simulink model "drembao_vel_torq"  (R2020b)
settings: Solver=VariableStepAuto  StartTime=0.0  StopTime=0.7998  FixedStep=dt  RelTol=1e-10  AbsTol=1e-14
values from neighbouring files (symbols this model uses):
  flux_initial = [1; 1]    [spmsm_param.m]    (also in spmsm_param_exp.m)
  G = [gamma, 0; 0, gamma]    [spmsm_param.m]    (also in spmsm_param_exp.m)
  gamma = 0.01    [spmsm_param.m]    (also in spmsm_param_exp.m = 50)
  gamma_L = 20000    [spmsm_param.m]    (also in spmsm_param_exp.m = 10000)
  gamma_w = 30000    [spmsm_param.m]    (also in spmsm_param_exp.m = 10000)
  I_d = 1    [spmsm_param.m]
  I_q = 1    [spmsm_param.m]
  I_w = 50    [spmsm_param.m]
  J = 59e-6    (= 5.9e-05)    [spmsm_param.m]    (also in spmsm_param_exp.m = 0.0015)
  L = 40.03e-3    (= 0.04003)    [spmsm_param.m]    (also in spmsm_param_exp.m = 0.0014)
  lm = 0.2086    [spmsm_param.m]    (also in spmsm_param_exp.m = 0.032)
  mu = 800    [spmsm_param.m]    (also in spmsm_param_exp.m = 100)
  np = 5    [spmsm_param.m]    (also in spmsm_param_exp.m = 8)
  nu = [50, 550]    [spmsm_param.m]    (also in spmsm_param_exp.m)
  P_d = 5    [spmsm_param.m]
  P_q = 5    [spmsm_param.m]
  P_w = 0.4    [spmsm_param.m]
  R = 8.875    [spmsm_param.m]    (also in spmsm_param_exp.m = 0.39)
  rho_1 = 0.9    [spmsm_param.m]    (also in spmsm_param_exp.m)
  S = [0, -1; 1, 0]    [spmsm_param.m]    (also in spmsm_param_exp.m)
  T = 2.0000e-04    (= 0.0002)    [prepare_timeseries_from_csv.m]
undefined symbols (not defined in the file or in its folder): j
libraries: pid_lib x3
settings Model: Creator=root  LastModifiedBy=R-1221
settings DataIOCC: ReturnWorkspaceOutputs=off
settings DebuggingCC: ArithmeticOperatorsInVariantConditions=warning
settings SFSimCC: SimUseLocalCustomCode=off  CustomCodeUndefinedFunction=UseInterfaceOnly
settings RTWCC: RTWUseLocalCustomCode=off

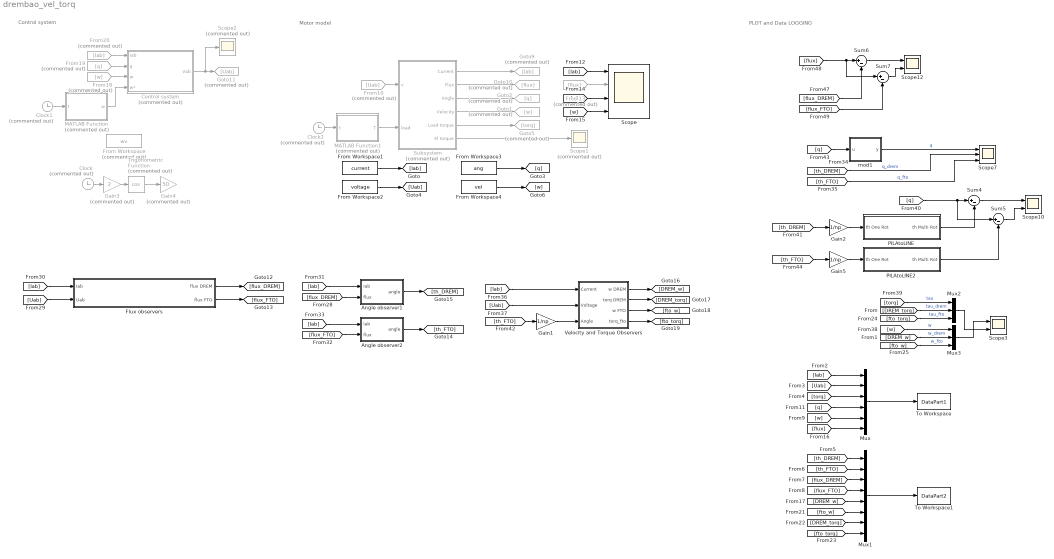
== system drembao_vel_torq ==
  note: PLOT and Data LOGGING
  note: Control system
  note: Motor model
  Angle observer1 : Subsystem
  Angle observer2 : Subsystem
  Clock : Clock  Commented=on
  Clock1 : Clock  Commented=on
  Clock2 : Clock  Commented=on
  Control system : Subsystem  Commented=on
  Flux observers : Subsystem
  From Workspace : FromWorkspace  Commented=on  VariableName=wv  SampleTime=-1
  From Workspace1 : FromWorkspace  VariableName=current  SampleTime=T
  From Workspace2 : FromWorkspace  VariableName=voltage  SampleTime=T
  From Workspace3 : FromWorkspace  VariableName=ang  SampleTime=T
  From Workspace4 : FromWorkspace  VariableName=vel  SampleTime=T
  From10 : From  Commented=on  GotoTag=Uab
  From13 : From  Commented=on  GotoTag=flux
  From18 : From  Commented=on  GotoTag=w
  From19 : From  Commented=on  GotoTag=q
  From20 : From  Commented=on  GotoTag=Iab
  Gain1 : Gain  Gain=1/np
  Gain2 : Gain  Gain=1/np
  Gain3 : Gain  Commented=on  Gain=2
  Gain4 : Gain  Commented=on  Gain=50
  Gain5 : Gain  Gain=1/np
  Goto1 : Goto  Commented=on  GotoTag=w
  Goto10 : Goto  Commented=on  GotoTag=flux
  Goto11 : Goto  Commented=on  GotoTag=Uab
  Goto2 : Goto  Commented=on  GotoTag=q
  Goto5 : Goto  Commented=on  GotoTag=torq
  Goto9 : Goto  Commented=on  GotoTag=Iab
  MATLAB Function : MATLAB Function  Commented=on  TreatAsAtomicUnit=on
  MATLAB Function1 : MATLAB Function  Commented=on  TreatAsAtomicUnit=on
  Mux : Mux  Inputs=6
  Mux1 : Mux  Inputs=8
  Mux2 : Mux  Inputs=3
  Mux3 : Mux  Inputs=3
  PILAtoLINE : Subsystem
  PILAtoLINE2 : Subsystem
  Scope : Scope  NumInputPorts=4
  Scope1 : Scope  Commented=on
  Scope10 : Scope  NumInputPorts=2
  Scope12 : Scope  NumInputPorts=2
  Scope2 : Scope  Commented=on
  Scope3 : Scope  NumInputPorts=2
  Scope7 : Scope  NumInputPorts=3
  Subsystem : Subsystem  Commented=on
  Sum{4..7} (4 alike) : Sum  Inputs=|+-
  To Workspace : ToWorkspace  VariableName=DataPart1  SaveFormat=Timeseries  SampleTime=-1
  To Workspace1 : ToWorkspace  VariableName=DataPart2  SaveFormat=Timeseries  SampleTime=-1
  Trigonometric Function : Trigonometry  Commented=on  Operator=cos
  Velocity and Torque Observers : Subsystem
  mod1 : MATLAB Function  TreatAsAtomicUnit=on
  wires:
  Subsystem/5(Load torque) -> Goto5/1
  Subsystem/2(Flux) -> Goto10/1
  Subsystem/1(Current) -> Goto9/1
  Subsystem/4(Velocity) -> Goto1/1
  Subsystem/3(Angle) -> Goto2/1
  Subsystem/6(El torque) -> Scope1/1
  From10/1 -> Subsystem/1(v)
  [Iab] -> Scope/1
  From13/1 -> Scope/2
  [q] -> Scope/3
  [w] -> Scope/4
  From18/1 -> Control system/3(w)
  MATLAB Function/1(w) -> Control system/4(w*)
  From19/1 -> Control system/2(q)
  From20/1 -> Control system/1(Iab)
  MATLAB Function1/1(T) -> Subsystem/2(load)
  Sum6/1 -> Scope12/1
  [flux] -> Sum7/1, Sum6/1
  [flux_DREM] -> Sum6/2
  [flux_FTO] -> Sum7/2
  Sum7/1 -> Scope12/2
  [Uab] -> Flux observers/2(Uab)
  [Iab] -> Flux observers/1(Iab)
  Flux observers/1(flux DREM) -> [flux_DREM]
  Flux observers/2(flux FTO) -> [flux_FTO]
  [q] -> mod1/1(u)
  [flux_DREM] -> Angle observer1/2(flux)
  [Iab] -> Angle observer1/1(Iab)
  Angle observer1/1(angle) -> [th_DREM]
  [Iab] -> Angle observer2/1(Iab)
  [flux_FTO] -> Angle observer2/2(flux)
  [th_FTO] -> Scope7/3  "q_fto"
  PILAtoLINE/1(th Multi Rot) -> Sum4/2
  [th_DREM] -> Gain2/1
  mod1/1(y) -> Scope7/1  "q"
  [th_DREM] -> Scope7/2  "q_drem"
  Angle observer2/1(angle) -> [th_FTO]
  [Uab] -> Velocity and Torque Observers/2(Voltage)
  Gain1/1 -> Velocity and Torque Observers/3(Angle)
  Velocity and Torque Observers/4(torq_fto) -> [fto_torq]
  [Iab] -> Velocity and Torque Observers/1(Current)
  Velocity and Torque Observers/3(w FTO) -> [fto_w]
  Velocity and Torque Observers/1(w DREM) -> [DREM_w]
  Velocity and Torque Observers/2(torq DREM) -> [DREM_torq]
  [th_FTO] -> Gain1/1
  Gain2/1 -> PILAtoLINE/1(th One Rot)
  [q] -> Sum5/1, Sum4/1
  Sum4/1 -> Scope10/1
  [th_FTO] -> Gain5/1
  Gain5/1 -> PILAtoLINE2/1(th One Rot)
  PILAtoLINE2/1(th Multi Rot) -> Sum5/2
  Sum5/1 -> Scope10/2
  Clock/1 -> Gain3/1
  Gain3/1 -> Trigonometric Function/1
  Trigonometric Function/1 -> Gain4/1
  [w] -> Mux3/1  "w"
  [DREM_w] -> Mux3/2  "w_drem"
  [DREM_torq] -> Mux2/2  "tau_drem"
  [torq] -> Mux2/1  "tau"
  [Iab] -> Mux/1
  [Uab] -> Mux/2
  [torq] -> Mux/3
  Mux/1 -> To Workspace/1
  [th_DREM] -> Mux1/1
  [th_FTO] -> Mux1/2
  [flux_DREM] -> Mux1/3
  [flux_FTO] -> Mux1/4
  Mux1/1 -> To Workspace1/1
  [q] -> Mux/4
  [w] -> Mux/5
  [flux] -> Mux/6
  [DREM_torq] -> Mux1/7
  [fto_w] -> Mux1/6
  [DREM_w] -> Mux1/5
  [fto_torq] -> Mux1/8
  Control system/1(Vab) -> Scope2/1, Goto11/1
  Clock1/1 -> MATLAB Function/1(t)
  Clock2/1 -> MATLAB Function1/1(t)
  From Workspace1/1 -> [Iab]
  From Workspace2/1 -> [Uab]
  From Workspace4/1 -> [w]
  From Workspace3/1 -> [q]
  [fto_torq] -> Mux2/3  "tau_fto"
  [fto_w] -> Mux3/3  "w_fto"
  Mux3/1 -> Scope3/1
  Mux2/1 -> Scope3/2

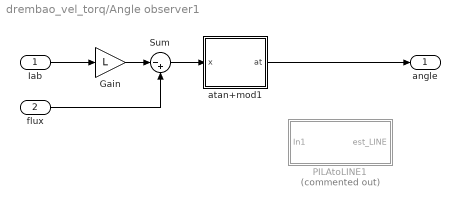
== system drembao_vel_torq/Angle observer1 ==
  Iab : Inport
  flux : Inport  Port=2
  Gain : Gain  Gain=L
  PILAtoLINE1 : Subsystem  Commented=on
  Sum : Sum  Inputs=|-+
  atan+mod1 : MATLAB Function  TreatAsAtomicUnit=on
  angle : Outport  VectorParamsAs1DForOutWhenUnconnected=off
  wires:
  Iab/1 -> Gain/1
  Gain/1 -> Sum/1
  flux/1 -> Sum/2
  Sum/1 -> atan+mod1/1(x)
  atan+mod1/1(at) -> angle/1

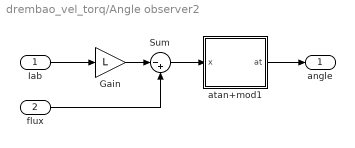
== system drembao_vel_torq/Angle observer2 ==
  Iab : Inport
  flux : Inport  Port=2
  Gain : Gain  Gain=L
  Sum : Sum  Inputs=|-+
  atan+mod1 : MATLAB Function  TreatAsAtomicUnit=on
  angle : Outport  VectorParamsAs1DForOutWhenUnconnected=off
  wires:
  Iab/1 -> Gain/1
  Gain/1 -> Sum/1
  flux/1 -> Sum/2
  Sum/1 -> atan+mod1/1(x)
  atan+mod1/1(at) -> angle/1

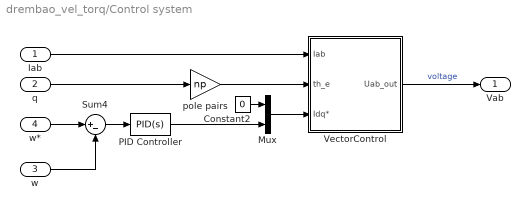
== system drembao_vel_torq/Control system ==
  Iab : Inport  PortDimensions=[2, 1]
  q : Inport  Port=2
  w : Inport  Port=3
  w* : Inport  Port=4
  Constant2 : Constant  Value=0
  Mux : Mux  Inputs=2
  PID Controller : pid_lib/PID Controller  Controller=PID  Form=Parallel  TimeDomain=Continuous-time  UseExternalTs=off  SampleTime=-1  IntegratorMethod=Forward Euler  FilterMethod=Forward Euler  ControllerParametersSource=internal  P=P_w  I=I_w  D=0  UseFilter=on  N=100  TunerSelectOption=Transfer Function Based (PID Tuner App)  InitialConditionSource=internal  InitialConditionForIntegrator=0  InitialConditionForFilter=0  DifferentiatorICPrevScaledInput=0  ExternalReset=none  TrackingMode=off  Kt=1  LimitOutput=off  SatLimitsSource=internal  UpperSaturationLimit=inf  LowerSaturationLimit=-inf  LinearizeAsGain=on  AntiWindupMode=none  Kb=1  POutMin=[]  POutMax=[]  IOutMin=[]  IOutMax=[]  DOutMin=[]  DOutMax=[]  NOutMin=[]  NOutMax=[]  SumOutMin=[]  SumOutMax=[]  SaturationOutMin=[]  SaturationOutMax=[]  PParamMin=[]  PParamMax=[]  IParamMin=[]  IParamMax=[]  DParamMin=[]  DParamMax=[]  NParamMin=[]  NParamMax=[]  KbParamMin=[]  KbParamMax=[]  KtParamMin=[]  KtParamMax=[]  KbOutMin=[]  KbOutMax=[]  KtOutMin=[]  KtOutMax=[]  IntegratorOutMin=[]  IntegratorOutMax=[]  FilterOutMin=[]  FilterOutMax=[]  SumI1OutMin=[]  SumI1OutMax=[]  SumI2OutMin=[]  SumI2OutMax=[]  SumI3OutMin=[]  SumI3OutMax=[]  SumI4OutMin=[]  SumI4OutMax=[]  SumDOutMin=[]  SumDOutMax=[]  DifferentiatorOutMin=[]  DifferentiatorOutMax=[]  FilterDiffOutCoefMin=[]  FilterDiffOutCoefMax=[]  ReciprocalOutMin=[]  ReciprocalOutMax=[]  SumDenOutMin=[]  SumDenOutMax=[]  SumNumOutMin=[]  SumNumOutMax=[]  DivideOutMin=[]  DivideOutMax=[]  UdiffTsProdOutMin=[]  UdiffTsProdOutMax=[]  NTsProdOutMin=[]  NTsProdOutMax=[]  UintegralTsProdOutMin=[]  UintegralTsProdOutMax=[]  UngainTsProdOutMin=[]  UngainTsProdOutMax=[]  IntegratorContinuousStateAttributes=''  IntegratorStateMustResolveToSignalObject=off  IntegratorRTWStateStorageClass=Auto  FilterContinuousStateAttributes=''  FilterStateMustResolveToSignalObject=off  FilterRTWStateStorageClass=Auto  ParallelPVariant=InternalParameters  IdealPVariant=Disabled  IVariant=InternalParameters  DVariant=InternalParameters  IntegratorVariant=Continuous  SatVariant=Disabled  AWVariant=Passthrough  PCopyVariant=Disabled  TRVariant=Disabled  FdbkBlocksVariant=Forward  IdealPFdbkVariant=Disabled  SatFdbkVariant=Disabled  DerivativeFilterVariant=ContFilter  NVariant=InternalParameters  NCopyVariant=Disabled  FilterICVariant=InternalICsFilter  IntegratorICVariant=InternalICs  ExternalResetVariant=Disabled  TRSumVariant=Passthrough  SumFdbkVariant=Disabled  SumVariant=Sum_PID  TsampFilterVariant=InternalTs  TsampNgainVariant=Passthrough  TsampIntegralVariant=Passthrough  ExternalSaturationOutDataTypeStr=Inherit: Same as second input
  Sum4 : Sum  Inputs=|+-
  VectorControl : Subsystem
  pole pairs : Gain  Gain=np
  Vab : Outport  PortDimensions=[2, 1]  VectorParamsAs1DForOutWhenUnconnected=off
  wires:
  w*/1 -> Sum4/1
  VectorControl/1(Uab_out) -> Vab/1  "voltage"
  w/1 -> Sum4/2
  Iab/1 -> VectorControl/1(Iab)
  Sum4/1 -> PID Controller/1
  q/1 -> pole pairs/1
  pole pairs/1 -> VectorControl/2(th_e)
  Mux/1 -> VectorControl/3(Idq*)
  PID Controller/1 -> Mux/2
  Constant2/1 -> Mux/1

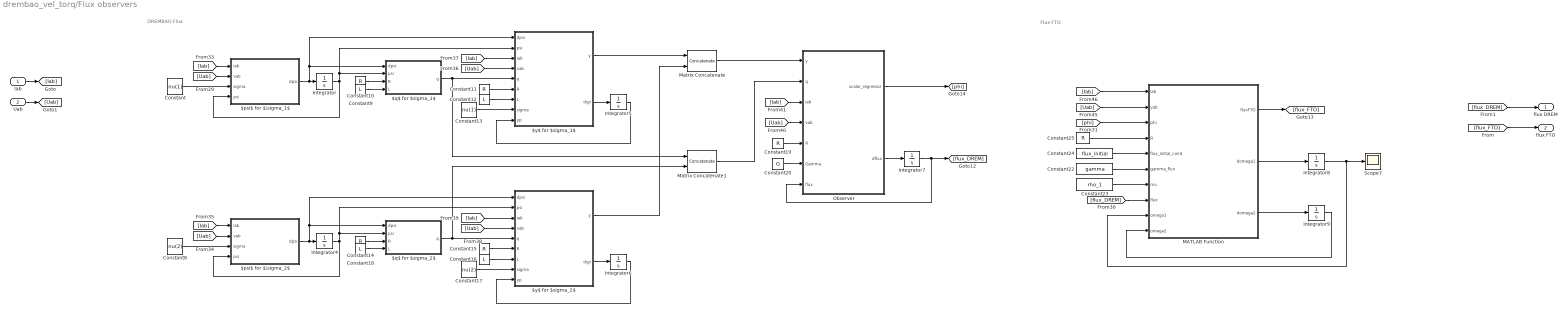
== system drembao_vel_torq/Flux observers ==
  note: Flux FTO
  note: DREMBAO Flux
  Iab : Inport
  Uab : Inport  Port=2
  $psi$ for $\sigma_1$ : MATLAB Function  TreatAsAtomicUnit=on
  $psi$ for $\sigma_2$ : MATLAB Function  TreatAsAtomicUnit=on
  $q$ for $sigma_1$ : MATLAB Function  TreatAsAtomicUnit=on
  $q$ for $sigma_2$ : MATLAB Function  TreatAsAtomicUnit=on
  $y$ for $sigma_1$ : MATLAB Function  TreatAsAtomicUnit=on
  $y$ for $sigma_2$ : MATLAB Function  TreatAsAtomicUnit=on
  Constant : Constant  Value=nu(1)
  Constant{10..11,14..15,19} (5 alike) : Constant  Value=R  VectorParams1D=off
  Constant{9,12,16,18} (4 alike) : Constant  Value=L  VectorParams1D=off
  Constant13 : Constant  Value=nu(1)
  Constant17 : Constant  Value=nu(2)
  Constant20 : Constant  Value=G  VectorParams1D=off
  Constant22 : Constant  Value=gamma
  Constant23 : Constant  Value=rho_1
  Constant24 : Constant  Value=flux_initial
  Constant25 : Constant  Value=R
  Constant8 : Constant  Value=nu(2)
  Integrator{,4..6,9} (5 alike) : Integrator
  Integrator7 : Integrator  InitialCondition=flux_initial
  Integrator8 : Integrator  InitialCondition=1
  MATLAB Function : MATLAB Function  TreatAsAtomicUnit=on
  Matrix Concatenate : Concatenate  Mode=Multidimensional array
  Matrix Concatenate1 : Concatenate  Mode=Multidimensional array
  Observer : MATLAB Function  TreatAsAtomicUnit=on
  Scope7 : Scope
  flux DREM : Outport  VectorParamsAs1DForOutWhenUnconnected=off
  flux FTO : Outport  Port=2  VectorParamsAs1DForOutWhenUnconnected=off
  wires:
  Constant22/1 -> MATLAB Function/6(gamma_flux)
  [Iab] -> $psi$ for $\sigma_1$/1(iab)
  $y$ for $sigma_1$/1(y) -> Matrix Concatenate/1
  Constant24/1 -> MATLAB Function/5(flux_initial_cond)
  Matrix Concatenate1/1 -> Observer/2(q)
  Matrix Concatenate/1 -> Observer/1(y)
  [Iab] -> MATLAB Function/1(iab)
  Constant10/1 -> $q$ for $sigma_1$/3(R)
  Constant8/1 -> $psi$ for $\sigma_2$/3(sigma)
  Integrator6/1 -> $y$ for $sigma_2$/9(yp)
  Constant/1 -> $psi$ for $\sigma_1$/3(sigma)
  Integrator8/1 -> Scope7/1, MATLAB Function/9(omega1)
  Constant19/1 -> Observer/5(R)
  Constant17/1 -> $y$ for $sigma_2$/8(sigma)
  Constant9/1 -> $q$ for $sigma_1$/4(L)
  Constant13/1 -> $y$ for $sigma_1$/8(sigma)
  [Uab] -> $y$ for $sigma_2$/4(vab)
  Integrator4/1 -> $q$ for $sigma_2$/2(psi), $y$ for $sigma_2$/2(psi), $psi$ for $\sigma_2$/4(psi)
  Integrator/1 -> $q$ for $sigma_1$/2(psi), $y$ for $sigma_1$/2(psi), $psi$ for $\sigma_1$/4(psi)
  Constant18/1 -> $q$ for $sigma_2$/4(L)
  Constant20/1 -> Observer/6(Gamma)
  [Uab] -> $psi$ for $\sigma_1$/2(vab)
  $y$ for $sigma_2$/2(dyp) -> Integrator6/1
  $psi$ for $\sigma_2$/1(dpsi) -> $q$ for $sigma_2$/1(dpsi), $y$ for $sigma_2$/1(dpsi), Integrator4/1
  Constant16/1 -> $y$ for $sigma_2$/7(L)
  $psi$ for $\sigma_1$/1(dpsi) -> $q$ for $sigma_1$/1(dpsi), $y$ for $sigma_1$/1(dpsi), Integrator/1
  Constant12/1 -> $y$ for $sigma_1$/7(L)
  Constant14/1 -> $q$ for $sigma_2$/3(R)
  Observer/2(dflux) -> Integrator7/1
  $y$ for $sigma_2$/1(y) -> Matrix Concatenate/2
  [Iab] -> Observer/3(iab)
  [Uab] -> MATLAB Function/2(vab)
  [Iab] -> $y$ for $sigma_2$/3(iab)
  Constant23/1 -> MATLAB Function/7(mu)
  $q$ for $sigma_2$/1(q) -> Matrix Concatenate1/2, $y$ for $sigma_2$/5(q)
  Constant25/1 -> MATLAB Function/4(R)
  Constant15/1 -> $y$ for $sigma_2$/6(R)
  [Uab] -> $psi$ for $\sigma_2$/2(vab)
  [Uab] -> Observer/4(vab)
  MATLAB Function/2(domega1) -> Integrator8/1
  Integrator9/1 -> MATLAB Function/10(omega2)
  [phi] -> MATLAB Function/3(phi)
  [Iab] -> $psi$ for $\sigma_2$/1(iab)
  [Uab] -> $y$ for $sigma_1$/4(vab)
  Constant11/1 -> $y$ for $sigma_1$/6(R)
  Integrator7/1 -> [flux_DREM], Observer/7(flux)
  MATLAB Function/3(domega2) -> Integrator9/1
  Observer/1(scalar_regressor) -> [phi]
  $q$ for $sigma_1$/1(q) -> Matrix Concatenate1/1, $y$ for $sigma_1$/5(q)
  MATLAB Function/1(fluxFTO) -> [flux_FTO]
  [flux_DREM] -> MATLAB Function/8(flux)
  [Iab] -> $y$ for $sigma_1$/3(iab)
  $y$ for $sigma_1$/2(dyp) -> Integrator5/1
  Integrator5/1 -> $y$ for $sigma_1$/9(yp)
  Iab/1 -> [Iab]
  Uab/1 -> [Uab]
  [flux_DREM] -> flux DREM/1
  [flux_FTO] -> flux FTO/1

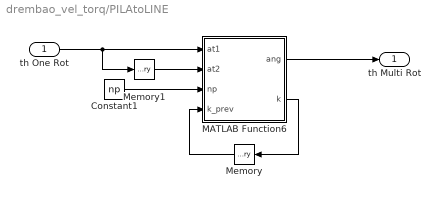
== system drembao_vel_torq/PILAtoLINE ==
  th One Rot : Inport
  Constant1 : Constant  Value=np
  MATLAB Function6 : MATLAB Function  TreatAsAtomicUnit=on
  Memory : Memory  InheritSampleTime=on  LinearizeMemory=on
  Memory1 : Memory  InheritSampleTime=on  LinearizeMemory=on
  th Multi Rot : Outport  VectorParamsAs1DForOutWhenUnconnected=off
  wires:
  MATLAB Function6/2(k) -> Memory/1
  Memory/1 -> MATLAB Function6/4(k_prev)
  Memory1/1 -> MATLAB Function6/2(at2)
  th One Rot/1 -> Memory1/1, MATLAB Function6/1(at1)
  Constant1/1 -> MATLAB Function6/3(np)
  MATLAB Function6/1(ang) -> th Multi Rot/1

== system drembao_vel_torq/PILAtoLINE2 ==
  th One Rot : Inport
  Constant1 : Constant  Value=np
  MATLAB Function6 : MATLAB Function  TreatAsAtomicUnit=on
  Memory : Memory  InheritSampleTime=on  LinearizeMemory=on
  Memory1 : Memory  InheritSampleTime=on  LinearizeMemory=on
  th Multi Rot : Outport  VectorParamsAs1DForOutWhenUnconnected=off
  wires:
  MATLAB Function6/2(k) -> Memory/1
  Memory/1 -> MATLAB Function6/4(k_prev)
  Memory1/1 -> MATLAB Function6/2(at2)
  th One Rot/1 -> Memory1/1, MATLAB Function6/1(at1)
  Constant1/1 -> MATLAB Function6/3(np)
  MATLAB Function6/1(ang) -> th Multi Rot/1

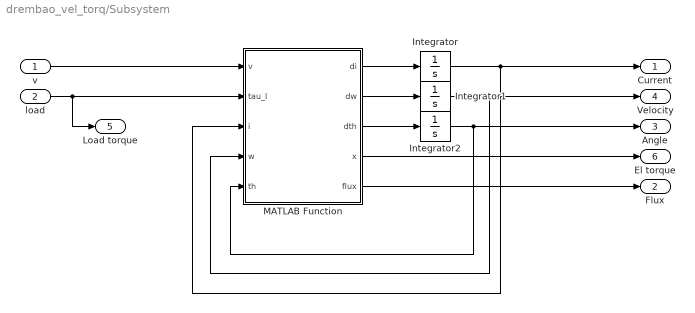
== system drembao_vel_torq/Subsystem ==
  v : Inport
  load : Inport  Port=2
  Integrator : Integrator
  Integrator1 : Integrator
  Integrator2 : Integrator
  MATLAB Function : MATLAB Function  TreatAsAtomicUnit=on
  Current : Outport  VectorParamsAs1DForOutWhenUnconnected=off
  Flux : Outport  Port=2  VectorParamsAs1DForOutWhenUnconnected=off
  Angle : Outport  Port=3  VectorParamsAs1DForOutWhenUnconnected=off
  Velocity : Outport  Port=4  VectorParamsAs1DForOutWhenUnconnected=off
  Load torque : Outport  Port=5  VectorParamsAs1DForOutWhenUnconnected=off
  El torque : Outport  Port=6  VectorParamsAs1DForOutWhenUnconnected=off
  wires:
  MATLAB Function/1(di) -> Integrator/1
  MATLAB Function/3(dth) -> Integrator2/1
  Integrator2/1 -> MATLAB Function/5(th), Angle/1
  Integrator/1 -> Current/1, MATLAB Function/3(i)
  MATLAB Function/2(dw) -> Integrator1/1
  load/1 -> Load torque/1, MATLAB Function/2(tau_l)
  v/1 -> MATLAB Function/1(v)
  Integrator1/1 -> Velocity/1, MATLAB Function/4(w)
  MATLAB Function/4(x) -> El torque/1
  MATLAB Function/5(flux) -> Flux/1

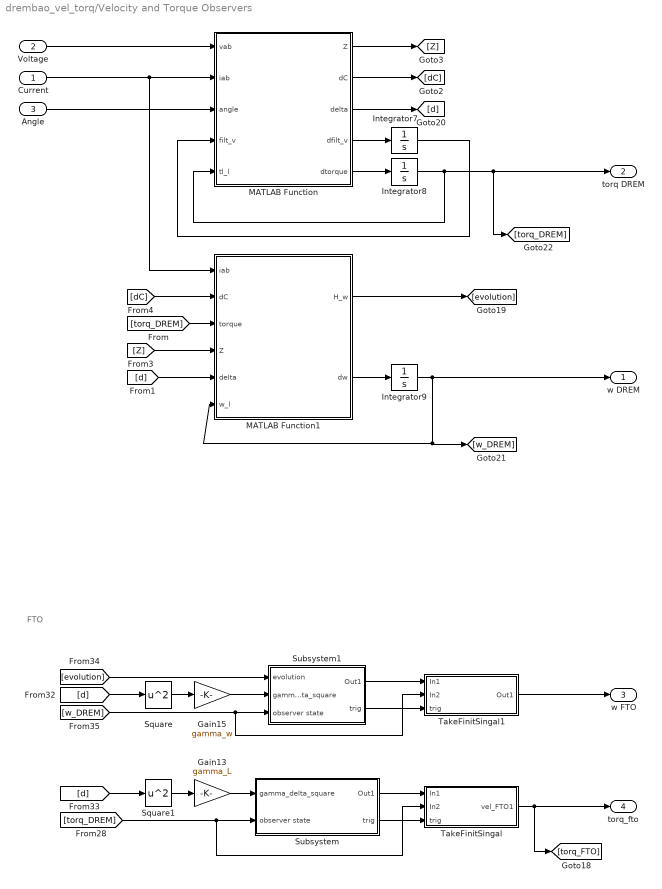
== system drembao_vel_torq/Velocity and Torque Observers ==
  note: FTO
  Current : Inport
  Voltage : Inport  Port=2
  Angle : Inport  Port=3
  Gain13 : Gain  Gain=gamma_L
  Gain15 : Gain  Gain=gamma_w
  Integrator7 : Integrator
  Integrator8 : Integrator  InitialCondition=0.01
  Integrator9 : Integrator  InitialCondition=1
  MATLAB Function : MATLAB Function  TreatAsAtomicUnit=on
  MATLAB Function1 : MATLAB Function  TreatAsAtomicUnit=on
  Square : Math  Operator=square  SignedPower=on  SaturateOnIntegerOverflow=on
  Square1 : Math  Operator=square  SignedPower=on  SaturateOnIntegerOverflow=on
  Subsystem : Subsystem
  Subsystem1 : Subsystem
  TakeFinitSingal : Subsystem
  TakeFinitSingal1 : Subsystem
  w DREM : Outport  VectorParamsAs1DForOutWhenUnconnected=off
  torq DREM : Outport  Port=2  VectorParamsAs1DForOutWhenUnconnected=off
  w FTO : Outport  Port=3  VectorParamsAs1DForOutWhenUnconnected=off
  torq_fto : Outport  Port=4  VectorParamsAs1DForOutWhenUnconnected=off
  wires:
  Square1/1 -> Gain13/1
  Gain13/1 -> Subsystem/1(gamma_delta_square)
  Subsystem/1(Out1) -> TakeFinitSingal/1(In1)
  TakeFinitSingal/1(vel_FTO1) -> [torq_FTO], torq_fto/1
  [torq_DREM] -> TakeFinitSingal/2(In2), Subsystem/2(observer state)
  Subsystem1/1(Out1) -> TakeFinitSingal1/1(In1)
  TakeFinitSingal1/1(Out1) -> w FTO/1
  Square/1 -> Gain15/1
  Gain15/1 -> Subsystem1/2(gamma_delta_square)
  Subsystem/2(trig) -> TakeFinitSingal/3(trig)
  Subsystem1/2(trig) -> TakeFinitSingal1/3(trig)
  MATLAB Function1/2(dw) -> Integrator9/1
  MATLAB Function/4(dfilt_v) -> Integrator7/1
  Integrator8/1 -> torq DREM/1, [torq_DREM], MATLAB Function/5(tl_l)
  MATLAB Function/5(dtorque) -> Integrator8/1
  Integrator9/1 -> w DREM/1, MATLAB Function1/6(w_l), [w_DREM]
  Integrator7/1 -> MATLAB Function/4(filt_v)
  Angle/1 -> MATLAB Function/3(angle)
  MATLAB Function/3(delta) -> [d]
  [d] -> Square/1
  [evolution] -> Subsystem1/1(evolution)
  [w_DREM] -> TakeFinitSingal1/2(In2), Subsystem1/3(observer state)
  [d] -> Square1/1
  Voltage/1 -> MATLAB Function/1(vab)
  [torq_DREM] -> MATLAB Function1/3(torque)
  [d] -> MATLAB Function1/5(delta)
  Current/1 -> MATLAB Function1/1(iab), MATLAB Function/2(iab)
  MATLAB Function/2(dC) -> [dC]
  MATLAB Function/1(Z) -> [Z]
  [Z] -> MATLAB Function1/4(Z)
  [dC] -> MATLAB Function1/2(dC)
  MATLAB Function1/1(H_w) -> [evolution]

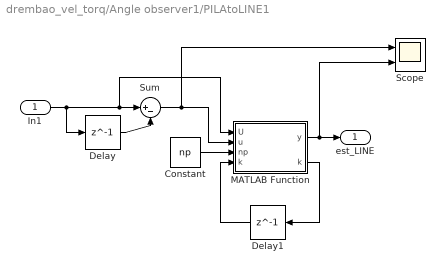
== system drembao_vel_torq/Angle observer1/PILAtoLINE1 ==
  In1 : Inport
  Constant : Constant  Value=np
  Delay : Delay  DelayLength=1  InitialCondition=0
  Delay1 : Delay  DelayLength=1  InitialCondition=0
  MATLAB Function : MATLAB Function  TreatAsAtomicUnit=on
  Scope : Scope  NumInputPorts=2
  Sum : Sum  Inputs=|+-
  est_LINE : Outport  VectorParamsAs1DForOutWhenUnconnected=off
  wires:
  Delay/1 -> Sum/2
  In1/1 -> Sum/1, MATLAB Function/1(U), Delay/1
  Sum/1 -> Scope/1, MATLAB Function/2(u)
  Constant/1 -> MATLAB Function/3(np)
  Delay1/1 -> MATLAB Function/4("k ")
  MATLAB Function/1(y) -> Scope/2, est_LINE/1
  MATLAB Function/2(k) -> Delay1/1

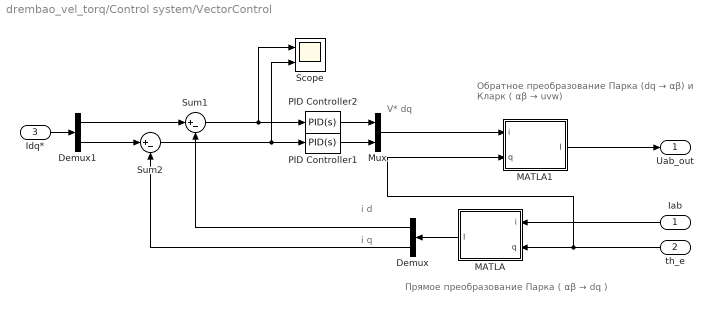
== system drembao_vel_torq/Control system/VectorControl ==
  note: V* dq
  note: i q
  note: i d
  note: Обратное преобразование
      | Парка (dq → αβ) и Кларк ( αβ → uvw)
  note: Прямое преобразование Парка ( αβ → dq )
  Iab : Inport
  th_e : Inport  Port=2
  Idq* : Inport  Port=3
  Demux : Demux  Outputs=2
  Demux1 : Demux  Outputs=2
  MATLA : MATLAB Function  TreatAsAtomicUnit=on
  MATLA1 : MATLAB Function  TreatAsAtomicUnit=on
  Mux : Mux  Inputs=2
  PID Controller1 : pid_lib/PID Controller  Controller=PID  Form=Parallel  TimeDomain=Continuous-time  UseExternalTs=off  SampleTime=-1  IntegratorMethod=Forward Euler  FilterMethod=Forward Euler  ControllerParametersSource=internal  P=P_q  I=I_q  D=0  UseFilter=on  N=100  TunerSelectOption=Transfer Function Based (PID Tuner App)  InitialConditionSource=internal  InitialConditionForIntegrator=0  InitialConditionForFilter=0  DifferentiatorICPrevScaledInput=0  ExternalReset=none  TrackingMode=off  Kt=1  LimitOutput=off  SatLimitsSource=internal  UpperSaturationLimit=inf  LowerSaturationLimit=-inf  LinearizeAsGain=on  AntiWindupMode=none  Kb=1  POutMin=[]  POutMax=[]  IOutMin=[]  IOutMax=[]  DOutMin=[]  DOutMax=[]  NOutMin=[]  NOutMax=[]  SumOutMin=[]  SumOutMax=[]  SaturationOutMin=[]  SaturationOutMax=[]  PParamMin=[]  PParamMax=[]  IParamMin=[]  IParamMax=[]  DParamMin=[]  DParamMax=[]  NParamMin=[]  NParamMax=[]  KbParamMin=[]  KbParamMax=[]  KtParamMin=[]  KtParamMax=[]  KbOutMin=[]  KbOutMax=[]  KtOutMin=[]  KtOutMax=[]  IntegratorOutMin=[]  IntegratorOutMax=[]  FilterOutMin=[]  FilterOutMax=[]  SumI1OutMin=[]  SumI1OutMax=[]  SumI2OutMin=[]  SumI2OutMax=[]  SumI3OutMin=[]  SumI3OutMax=[]  SumI4OutMin=[]  SumI4OutMax=[]  SumDOutMin=[]  SumDOutMax=[]  DifferentiatorOutMin=[]  DifferentiatorOutMax=[]  FilterDiffOutCoefMin=[]  FilterDiffOutCoefMax=[]  ReciprocalOutMin=[]  ReciprocalOutMax=[]  SumDenOutMin=[]  SumDenOutMax=[]  SumNumOutMin=[]  SumNumOutMax=[]  DivideOutMin=[]  DivideOutMax=[]  UdiffTsProdOutMin=[]  UdiffTsProdOutMax=[]  NTsProdOutMin=[]  NTsProdOutMax=[]  UintegralTsProdOutMin=[]  UintegralTsProdOutMax=[]  UngainTsProdOutMin=[]  UngainTsProdOutMax=[]  IntegratorContinuousStateAttributes=''  IntegratorStateMustResolveToSignalObject=off  IntegratorRTWStateStorageClass=Auto  FilterContinuousStateAttributes=''  FilterStateMustResolveToSignalObject=off  FilterRTWStateStorageClass=Auto  ParallelPVariant=InternalParameters  IdealPVariant=Disabled  IVariant=InternalParameters  DVariant=InternalParameters  IntegratorVariant=Continuous  SatVariant=Disabled  AWVariant=Passthrough  PCopyVariant=Disabled  TRVariant=Disabled  FdbkBlocksVariant=Forward  IdealPFdbkVariant=Disabled  SatFdbkVariant=Disabled  DerivativeFilterVariant=ContFilter  NVariant=InternalParameters  NCopyVariant=Disabled  FilterICVariant=InternalICsFilter  IntegratorICVariant=InternalICs  ExternalResetVariant=Disabled  TRSumVariant=Passthrough  SumFdbkVariant=Disabled  SumVariant=Sum_PID  TsampFilterVariant=InternalTs  TsampNgainVariant=Passthrough  TsampIntegralVariant=Passthrough  ExternalSaturationOutDataTypeStr=Inherit: Same as second input
  PID Controller2 : pid_lib/PID Controller  Controller=PID  Form=Parallel  TimeDomain=Continuous-time  UseExternalTs=off  SampleTime=-1  IntegratorMethod=Forward Euler  FilterMethod=Forward Euler  ControllerParametersSource=internal  P=P_d  I=I_d  D=0  UseFilter=on  N=100  TunerSelectOption=Transfer Function Based (PID Tuner App)  InitialConditionSource=internal  InitialConditionForIntegrator=0  InitialConditionForFilter=0  DifferentiatorICPrevScaledInput=0  ExternalReset=none  TrackingMode=off  Kt=1  LimitOutput=off  SatLimitsSource=internal  UpperSaturationLimit=inf  LowerSaturationLimit=-inf  LinearizeAsGain=on  AntiWindupMode=none  Kb=1  POutMin=[]  POutMax=[]  IOutMin=[]  IOutMax=[]  DOutMin=[]  DOutMax=[]  NOutMin=[]  NOutMax=[]  SumOutMin=[]  SumOutMax=[]  SaturationOutMin=[]  SaturationOutMax=[]  PParamMin=[]  PParamMax=[]  IParamMin=[]  IParamMax=[]  DParamMin=[]  DParamMax=[]  NParamMin=[]  NParamMax=[]  KbParamMin=[]  KbParamMax=[]  KtParamMin=[]  KtParamMax=[]  KbOutMin=[]  KbOutMax=[]  KtOutMin=[]  KtOutMax=[]  IntegratorOutMin=[]  IntegratorOutMax=[]  FilterOutMin=[]  FilterOutMax=[]  SumI1OutMin=[]  SumI1OutMax=[]  SumI2OutMin=[]  SumI2OutMax=[]  SumI3OutMin=[]  SumI3OutMax=[]  SumI4OutMin=[]  SumI4OutMax=[]  SumDOutMin=[]  SumDOutMax=[]  DifferentiatorOutMin=[]  DifferentiatorOutMax=[]  FilterDiffOutCoefMin=[]  FilterDiffOutCoefMax=[]  ReciprocalOutMin=[]  ReciprocalOutMax=[]  SumDenOutMin=[]  SumDenOutMax=[]  SumNumOutMin=[]  SumNumOutMax=[]  DivideOutMin=[]  DivideOutMax=[]  UdiffTsProdOutMin=[]  UdiffTsProdOutMax=[]  NTsProdOutMin=[]  NTsProdOutMax=[]  UintegralTsProdOutMin=[]  UintegralTsProdOutMax=[]  UngainTsProdOutMin=[]  UngainTsProdOutMax=[]  IntegratorContinuousStateAttributes=''  IntegratorStateMustResolveToSignalObject=off  IntegratorRTWStateStorageClass=Auto  FilterContinuousStateAttributes=''  FilterStateMustResolveToSignalObject=off  FilterRTWStateStorageClass=Auto  ParallelPVariant=InternalParameters  IdealPVariant=Disabled  IVariant=InternalParameters  DVariant=InternalParameters  IntegratorVariant=Continuous  SatVariant=Disabled  AWVariant=Passthrough  PCopyVariant=Disabled  TRVariant=Disabled  FdbkBlocksVariant=Forward  IdealPFdbkVariant=Disabled  SatFdbkVariant=Disabled  DerivativeFilterVariant=ContFilter  NVariant=InternalParameters  NCopyVariant=Disabled  FilterICVariant=InternalICsFilter  IntegratorICVariant=InternalICs  ExternalResetVariant=Disabled  TRSumVariant=Passthrough  SumFdbkVariant=Disabled  SumVariant=Sum_PID  TsampFilterVariant=InternalTs  TsampNgainVariant=Passthrough  TsampIntegralVariant=Passthrough  ExternalSaturationOutDataTypeStr=Inherit: Same as second input
  Scope : Scope  NumInputPorts=2
  Sum1 : Sum  Inputs=|+-
  Sum2 : Sum  Inputs=|+-
  Uab_out : Outport  VectorParamsAs1DForOutWhenUnconnected=off
  wires:
  PID Controller2/1 -> Mux/1
  Iab/1 -> MATLA/1(i)
  PID Controller1/1 -> Mux/2
  MATLA/1(I) -> Demux/1
  MATLA1/1(I) -> Uab_out/1
  Demux1/1 -> Sum1/1
  th_e/1 -> MATLA1/2(q), MATLA/2(q)
  Demux/1 -> Sum1/2
  Demux/2 -> Sum2/2
  Sum2/1 -> Scope/2, PID Controller1/1
  Sum1/1 -> Scope/1, PID Controller2/1
  Mux/1 -> MATLA1/1(i)
  Idq*/1 -> Demux1/1
  Demux1/2 -> Sum2/1

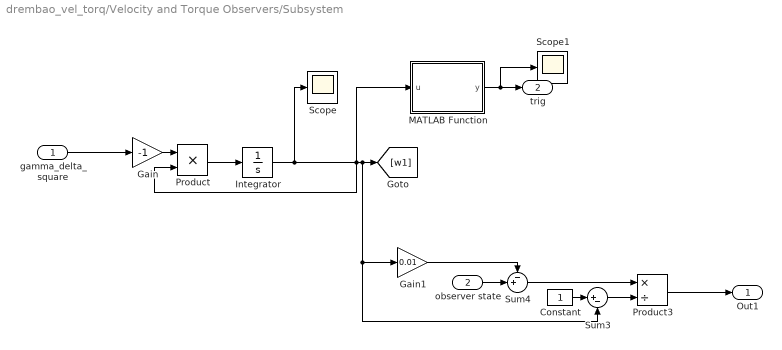
== system drembao_vel_torq/Velocity and Torque Observers/Subsystem ==
  gamma_delta_square : Inport
  observer state : Inport  Port=2
  Constant : Constant
  Gain : Gain  Gain=-1
  Gain1 : Gain  Gain=0.01
  Integrator : Integrator  InitialCondition=1
  MATLAB Function : MATLAB Function  TreatAsAtomicUnit=on
  Product : Product
  Product3 : Product  Inputs=*/
  Scope : Scope
  Scope1 : Scope
  Sum3 : Sum  Inputs=|+-
  Sum4 : Sum  Inputs=-+|
  Out1 : Outport  VectorParamsAs1DForOutWhenUnconnected=off
  trig : Outport  Port=2  VectorParamsAs1DForOutWhenUnconnected=off
  wires:
  gamma_delta_square/1 -> Gain/1
  Gain/1 -> Product/1
  Product/1 -> Integrator/1
  Constant/1 -> Sum3/1
  Product3/1 -> Out1/1
  Sum3/1 -> Product3/2
  observer state/1 -> Sum4/2
  Sum4/1 -> Product3/1
  MATLAB Function/1(y) -> Scope1/1, trig/1
  Integrator/1 -> Scope/1, MATLAB Function/1(u), Product/2, Sum3/2, Gain1/1, [w1]
  Gain1/1 -> Sum4/1

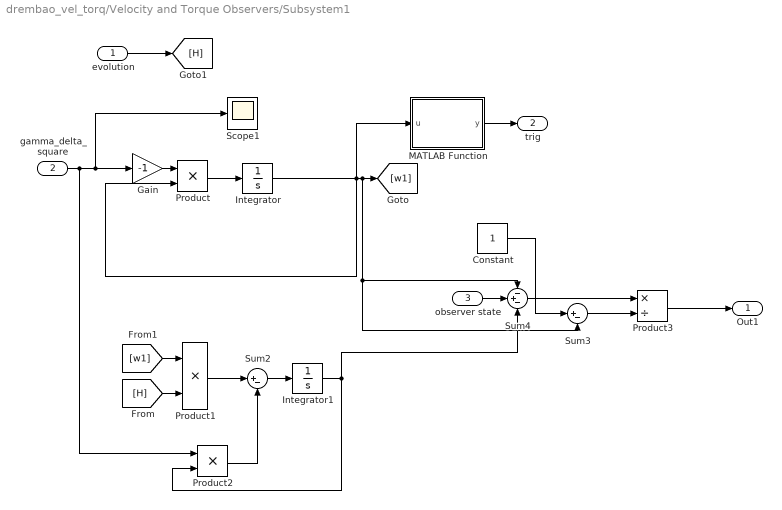
== system drembao_vel_torq/Velocity and Torque Observers/Subsystem1 ==
  evolution : Inport
  gamma_delta_square : Inport  Port=2
  observer state : Inport  Port=3
  Constant : Constant
  Gain : Gain  Gain=-1
  Integrator : Integrator  InitialCondition=1
  Integrator1 : Integrator
  MATLAB Function : MATLAB Function  TreatAsAtomicUnit=on
  Product : Product
  Product1 : Product
  Product2 : Product
  Product3 : Product  Inputs=*/
  Scope1 : Scope
  Sum2 : Sum  Inputs=|+-
  Sum3 : Sum  Inputs=|+-
  Sum4 : Sum  Inputs=-+-
  Out1 : Outport  VectorParamsAs1DForOutWhenUnconnected=off
  trig : Outport  Port=2  VectorParamsAs1DForOutWhenUnconnected=off
  wires:
  gamma_delta_square/1 -> Product2/1, Scope1/1, Gain/1
  Gain/1 -> Product/1
  Integrator/1 -> MATLAB Function/1(u), Product/2, Sum4/1, Sum3/2, [w1]
  Product/1 -> Integrator/1
  Constant/1 -> Sum3/1
  [w1] -> Product1/1
  [H] -> Product1/2
  Product1/1 -> Sum2/1
  Product2/1 -> Sum2/2
  Sum2/1 -> Integrator1/1
  Integrator1/1 -> Sum4/3, Product2/2
  Product3/1 -> Out1/1
  Sum3/1 -> Product3/2
  observer state/1 -> Sum4/2
  Sum4/1 -> Product3/1
  evolution/1 -> [H]
  MATLAB Function/1(y) -> trig/1

== system drembao_vel_torq/Velocity and Torque Observers/TakeFinitSingal ==
  In1 : Inport
  In2 : Inport  Port=2
  trig : Inport  Port=3
  Switch : Switch  Criteria=u2 > Threshold
  vel_FTO1 : Outport  VectorParamsAs1DForOutWhenUnconnected=off
  wires:
  In1/1 -> Switch/1
  In2/1 -> Switch/3
  Switch/1 -> vel_FTO1/1
  trig/1 -> Switch/2

== system drembao_vel_torq/Velocity and Torque Observers/TakeFinitSingal1 ==
  In1 : Inport
  In2 : Inport  Port=2
  trig : Inport  Port=3
  Switch : Switch  Criteria=u2 > Threshold
  Out1 : Outport  VectorParamsAs1DForOutWhenUnconnected=off
  wires:
  In1/1 -> Switch/1
  In2/1 -> Switch/3
  Switch/1 -> Out1/1
  trig/1 -> Switch/2

== matlab function drembao_vel_torq/Subsystem/MATLAB Function ==
  data: v input size=[2, 1]; tau_l input size=1; di output size=[2, 1]; i input size=[2, 1]; w input size=1; th input size=1; dw output size=1; dth output size=1; R parameter; S parameter; np parameter; j parameter; L parameter; lm parameter; x output; flux output
function [di, dw, dth, x, flux] = SPMSM_m(v, tau_l, i, w, th, R, S, np, j, L, lm)

    C = [cos(np*th); sin(np*th)];
    dC = np*S*C;
    di = 1/L * (v - R*i - lm*w*dC);

    % Total torque with acceleration
    T = lm*i'*dC - tau_l;
    dw = 1/j * T;

    dth = w;
    x = T; %lm*C;
    flux = L*i + lm*C;

end

== matlab function drembao_vel_torq/Flux observers/$psi$ for $\sigma_1$ ==
  data: iab input; vab input; sigma input; psi input; dpsi output
function dpsi = PSI(iab, vab, sigma, psi)
    dpsi = -sigma*psi + sigma*[iab', vab', iab'*iab, vab'*iab];
end

== matlab function drembao_vel_torq/Flux observers/$psi$ for $\sigma_2$ ==
  data: iab input; vab input; sigma input; psi input; dpsi output
function dpsi = PSI(iab, vab, sigma, psi)
    dpsi = -sigma*psi + sigma*[iab', vab', iab'*iab, vab'*iab];
end

== matlab function drembao_vel_torq/Flux observers/$q$ for $sigma_1$ ==
  data: dpsi input; psi input; q output; R input; L input
function q = Q(dpsi, psi, R, L)

    q = psi(:, 3:4) - L*dpsi(:, 1:2) - R*psi(:, 1:2);

end

== matlab function drembao_vel_torq/Control system/VectorControl/MATLA ==
  data: i input; I output; q input
function I = DirParke(i, q)

    I = [cos(q), sin(q); -sin(q), cos(q)]*[i(1); i(2)];

== matlab function drembao_vel_torq/Control system/VectorControl/MATLA1 ==
  data: i input; I output; q input
function I = InvParke(i, q)

    I = [cos(q), -sin(q); sin(q), cos(q)]*[i(1); i(2)];

== matlab function drembao_vel_torq/Flux observers/$y$ for $sigma_1$ ==
  data: dpsi input; psi input; iab input; y output; vab input; q input; R input; L input; sigma input; yp input; dyp output
function [y, dyp] = Yp(dpsi, psi, iab, vab, q, R, L, sigma, yp)

    dyp = -sigma*yp + q*(vab - R*iab);
    y = yp - 1/2*L^2*dpsi(:, 5) + L*psi(:, 6) - R*L*psi(:, 5);

end

== matlab function drembao_vel_torq/Flux observers/$q$ for $sigma_2$ ==
  data: dpsi input; psi input; q output; R input; L input
function q = Q(dpsi, psi, R, L)

    q = psi(:, 3:4) - L*dpsi(:, 1:2) - R*psi(:, 1:2);

end

== matlab function drembao_vel_torq/Flux observers/$y$ for $sigma_2$ ==
  data: dpsi input; psi input; iab input; y output; vab input; q input; R input; L input; sigma input; yp input; dyp output
function [y, dyp] = Yp(dpsi, psi, iab, vab, q, R, L, sigma, yp)

    dyp = -sigma*yp + q*(vab - R*iab);
    y = yp - 1/2*L^2*dpsi(:, 5) + L*psi(:, 6) - R*L*psi(:, 5);

end

== matlab function drembao_vel_torq/Flux observers/Observer ==
  data: scalar_regressor output; y input; q input; iab input; dflux output; vab input; R input; Gamma input; flux input
function [scalar_regressor, dflux] = Observer(y, q, iab, vab, R, Gamma, flux)

	adjq = zeros(size(q));
    p = 1:length(q);
    [s1, s2] = size(q);
    
    for i = 1:s1
        for j = 1:s2
            minor = q(setdiff(p, i), setdiff(p, j));
            adjq(j, i) = (-1)^(i + j)*det(minor);
        end
    end

    phi = det(q);
    xi = adjq*y;

    scalar_regressor = phi;
    dflux = vab - R*iab + Gamma*phi*(xi - phi*flux);

end

== matlab function drembao_vel_torq/Angle observer1/atan+mod1 ==
  data: x input; at output
function at = atan2pi(x)

    at = atan2(x(2), x(1));
    at = mod(at, 2*pi);

end

== matlab function drembao_vel_torq/mod1 ==
  data: u input; y output; np parameter
function y = fcn(u, np)

    y = mod(np*u, 2*pi);

end

== matlab function drembao_vel_torq/Flux observers/MATLAB Function ==
  data: fluxFTO output; iab input; vab input; phi input; R input; flux_initial_cond input; gamma_flux input; mu input; flux input; domega1 output; omega1 input; domega2 output; omega2 input
function [fluxFTO, domega1, domega2] = fluxFTO(iab, vab, phi, R, flux_initial_cond, gamma_flux, mu, flux, omega1, omega2)

    domega1 = -gamma_flux*phi^2*omega1;
    domega2 = -gamma_flux*phi^2*omega2 + (vab - R*iab)*omega1;

    clip = omega1;
    if (clip > mu)
        clip = mu;
    end

    fluxFTO = (flux - flux_initial_cond*clip - omega2)/(1 - clip);

end

== matlab function drembao_vel_torq/PILAtoLINE/MATLAB Function6 ==
  data: at1 input; ang output; at2 input; np input; k_prev input; k output
function [ang, k] = wrapPhase(at1, at2, np, k_prev)

    diff = at1 - at2;
    k = k_prev;
    if diff + 1.7*pi/np < 0 
        k = k_prev + 1;
    elseif diff - 1.7*pi/np > 0
        k = k_prev - 1;
    end

    ang = at1 + 2*pi/np * k;

end

== matlab function drembao_vel_torq/Velocity and Torque Observers/Subsystem/MATLAB Function ==
  data: u input; y output; rho_2 parameter
function y = fcn(u, rho_2)
if u < rho_2
    y = 1;
else y = 0;
end

== matlab function drembao_vel_torq/Velocity and Torque Observers/MATLAB Function ==
  data: Z output; dC output; delta output; dfilt_v output; dtorque output; vab input; iab input; angle input; filt_v input size=[10, 1]; tl_l input; np parameter; S parameter; mu parameter; J parameter; gamma_L parameter; lm parameter; L parameter; R parameter
function [Z, dC, delta, dfilt_v, dtorque] = DREMBAO_TL(vab, iab, angle, filt_v, tl_l, np, S, mu, J, gamma_L, lm, L, R)

    C = [cos(np*angle); sin(np*angle)];
    dC = -lm*np*S*C;
    c = iab*R - vab;
    tq1 = filt_v(1:2);
    q2 = filt_v(3:4);
    fc = filt_v(5:6);
    tfpi = filt_v(7:8);
    tff = filt_v(9:10);

    dq2 = mu*(dC - q2);
    q1 = tq1/J;
    tq1 = q2 - mu*tq1;
    dfc = mu*(c - fc);
    tfpi = (iab - tfpi)*mu;fpi = tfpi * L;
    ff = tff/J;
    tff = (iab'*dC*q2 - tff*mu);

    z = fpi + fc - ff;
    Q = [q1, q2];
    delta = det(Q);
    adjQ = [Q(2, 2), -Q(1, 2); -Q(2, 1), Q(1, 1)];
    Z = adjQ * z;
    dtorque = (Z(1) - tl_l*delta)*gamma_L*delta;
    dfilt_v = [tq1; dq2; dfc; tfpi; tff];

end

== matlab function drembao_vel_torq/Velocity and Torque Observers/Subsystem1/MATLAB Function ==
  data: u input; y output; rho_3 parameter
function y = fcn(u, rho_3)
if u < rho_3
    y = 1;
else
    y = 0;
end

== matlab function drembao_vel_torq/Velocity and Torque Observers/MATLAB Function1 ==
  data: H_w output; iab input; dC input; torque input; Z input; J parameter; gamma_w parameter; delta input; dw output; w_l input
function [H_w, dw] = DREMBAO_W(iab, dC, torque, Z, J, gamma_w, delta, w_l)
    H_w = -(torque + iab'*dC)/J;
    dw = delta*gamma_w*(Z(2) - w_l * delta) + H_w;
end

== matlab function drembao_vel_torq/MATLAB Function ==
  data: t input; w output
function w = VEL_FUNC(t)

    w = 20;
    
    if (t > 0.2)
        w = 30;
    end

    if (t > 0.4)
        w = 40;
    end

    if (t > 0.6)
        w = 50;
    end

    if (t > 0.8)
        w = 60;
    end

end

== matlab function drembao_vel_torq/MATLAB Function1 ==
  data: t input; T output
function T = TORQ_FUNC(t)

    T = 0.05*floor(t*10) + 0.1;

end

== matlab function drembao_vel_torq/Angle observer2/atan+mod1 ==
  data: x input; at output
function at = atan2pi(x)

    at = atan2(x(2), x(1));
    at = mod(at, 2*pi);

end

== matlab function drembao_vel_torq/Angle observer1/PILAtoLINE1/MATLAB Function ==
  data: U input; u input; y output; np input; k input; k output
function [y,k] = fcn(U,u,np, k)
if abs(u)- pi/np > 0
    if u > 0
        k = k - 1;
    else
        k = k + 1; 
    end 
end
y = U + k*2*pi/np;
end

== matlab function drembao_vel_torq/PILAtoLINE2/MATLAB Function6 ==
  data: at1 input; ang output; at2 input; np input; k_prev input; k output
function [ang, k] = wrapPhase(at1, at2, np, k_prev)

    diff = at1 - at2;
    k = k_prev;
    if diff + 1.7*pi/np < 0 
        k = k_prev + 1;
    elseif diff - 1.7*pi/np > 0
        k = k_prev - 1;
    end

    ang = at1 + 2*pi/np * k;

end
